simulink model "MASTER"  (R2019a)
settings: Solver=FixedStepAuto  StartTime=0.0  StopTime=10.0  FixedStep=0.001  RelTol=1e-3
PreLoadFcn:
  | waijung.modelPreload; % Required for working with Waijung Blockset. Do not remove.
undefined symbols (not defined in the file): HSEOSC, Link, LQFP100, ST, STM32F407VG
libraries: simulink x17, stm32f4_canbus_lib x7, stm32f4_tim_lib x1, stm32f4_io_lib x1, stm32f4_device_config_lib x1
(part 1 of 2)
CloseFcn:
  | waijung.modelClose; % Required for working with Waijung Blockset. Do not remove.
settings Model: Creator=Le Thanh Tu  LastModifiedBy=Le Thanh Tu
settings OptimizationCC: DefaultParameterBehavior=Inlined  PassReuseOutputArgsAs=Individual arguments
settings DebuggingCC: ParameterTunabilityLossMsg=error
settings HardwareCC: ProdBitPerPointer=32  ProdBitPerSizeT=32  ProdBitPerPtrDiffT=32  ProdLargestAtomicFloat=None  ProdIntDivRoundTo=Undefined  ProdWordSize=32  ProdHWDeviceType=ARM Compatible->Cortex - M4  TargetEndianess=LittleEndian  TargetHWDeviceType=ARM Compatible->Cortex - M4
settings SFSimCC: MATLABDynamicMemAlloc=off
settings RTWCC: SystemTargetFile=stm32f4.tlc  GenerateMakefile=off  TemplateMakefile=ert_default_tmf  Description=STM32F4 Target  GenerateReport=on  IncludeHyperlinkInReport=on  LaunchReport=on  GenerateTraceInfo=on  GenerateTraceReport=on  GenerateTraceReportSl=on  GenerateTraceReportSf=on  GenerateTraceReportEml=on
settings CodeAppCC: ForceParamTrailComments=on  IgnoreCustomStorageClasses=off  OperatorAnnotations=on  SimulinkDataObjDesc=on  SFDataObjDesc=on  InsertBlockDesc=on
settings STFCustomTargetCC: MultiwordLength=256  ModelReferenceCompliant=off  CombineOutputUpdateFcns=on  ERTCustomFileBanners=on  SupportNonInlinedSFcns=off  RemoveResetFunc=on  SupportVariableSizeSignals=on  MATLABClassNameForMDSCustomization=Simulink.SoftwareTarget.ERTCustomization  GRTInterface=off  SystemTargetFile=stm32f4.tlc
settings ERTTargetCC: ModelReferenceCompliant=off  ParMdlRefBuildCompliant=off  CompOptLevelCompliant=off  ConcurrentExecutionCompliant=off  SupportContinuousTime=on  SupportVariableSizeSignals=on  ModelStepFunctionPrototypeControlCompliant=off  CPPClassGenCompliant=off  UseToolchainInfoCompliant=off  InlinedParameterPlacement=NonHierarchical  ERTSrcFileBannerTemplate=stm32f4_code_template.cgt  ERTHdrFileBannerTemplate=stm32f4_code_template.cgt  ERTDataSrcFileTemplate=stm32f4_code_template.cgt  ERTDataHdrFileTemplate=stm32f4_code_template.cgt  ERTCustomFileTemplate=stm32f4_file_process.tlc

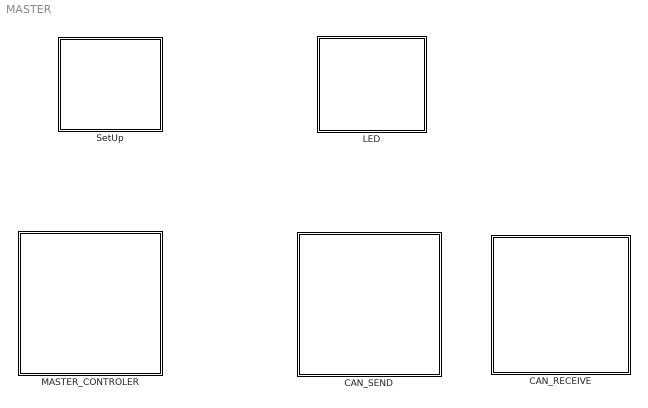
== system MASTER ==
  CAN_RECEIVE : Subsystem
  CAN_SEND : Subsystem
  LED : Subsystem
  MASTER_CONTROLER : Subsystem
  SetUp : Subsystem

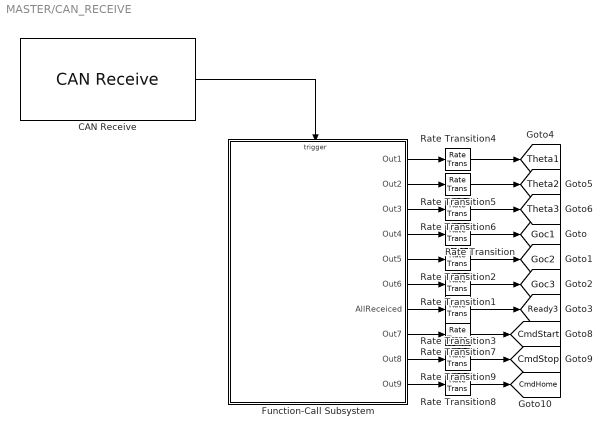
== system MASTER/CAN_RECEIVE ==
  CAN Receive : stm32f4_canbus_lib/CAN Receive  conf=Rx  canmodule=1  idtype=Standard  filtertype=Mask  id=0  idmask=0  enableisr=on  usedlc=off  datatype=single  data0type=uint32  data1type=uint32  data2type=Not used  data3type=Not used  data4type=Not used  data5type=Not used  data6type=Not used  data7type=Not used  buffersize=8  sampletime=-1  sampletimestr=-1  blockid=CAN_RECEIVECANReceive  inputarray=[]  inputlabelarray={}  outputarray=[7]  outputlabelarray={'Call ISR' }  compat=0  confstr="[\"Standard\",\"Mask\",\"0\",\"0\",\"off\",\"uint32\",\"uint32\",\"Not used\",\"Not used\",\"Not used\",\"Not used\",\"Not used\",\"Not used\",\"8\",\"0\",\"0\",\"0\",\"4\"]"
      settings: SourceProductName=Waijung Blockset
  Function-Call Subsystem : Subsystem  TreatAsAtomicUnit=on
  Rate Transition{,1..9} (10 alike) : RateTransition  Deterministic=off
  tag scope: CmdHome=global, CmdStart=global, CmdStop=global, Goc1=global, Goc2=global, Goc3=global, Ready3=global, Theta1=global, Theta2=global, Theta3=global
  wires:
  Function-Call Subsystem/7(AllReceiced) -> Rate Transition3/1
  Rate Transition2/1 -> [Goc2]
  Function-Call Subsystem/8(Out7) -> Rate Transition7/1
  Rate Transition1/1 -> [Goc3]
  CAN Receive/1 -> Function-Call Subsystem/Trigger
  Rate Transition/1 -> [Goc1]
  Rate Transition9/1 -> [CmdStop]
  Function-Call Subsystem/10(Out9) -> Rate Transition8/1
  Function-Call Subsystem/3(Out3) -> Rate Transition6/1
  Function-Call Subsystem/2(Out2) -> Rate Transition5/1
  Function-Call Subsystem/4(Out4) -> Rate Transition/1
  Rate Transition7/1 -> [CmdStart]
  Function-Call Subsystem/6(Out6) -> Rate Transition1/1
  Rate Transition6/1 -> [Theta3]
  Rate Transition3/1 -> [Ready3]
  Function-Call Subsystem/9(Out8) -> Rate Transition9/1
  Function-Call Subsystem/5(Out5) -> Rate Transition2/1
  Rate Transition8/1 -> [CmdHome]
  Rate Transition4/1 -> [Theta1]
  Rate Transition5/1 -> [Theta2]
  Function-Call Subsystem/1(Out1) -> Rate Transition4/1

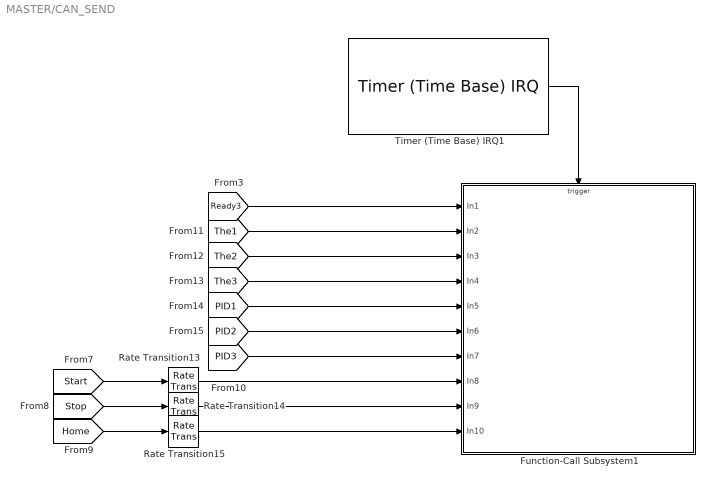
== system MASTER/CAN_SEND ==
  Function-Call Subsystem1 : Subsystem  TreatAsAtomicUnit=on
  Rate Transition13 : RateTransition  Deterministic=off
  Rate Transition14 : RateTransition  Deterministic=off
  Rate Transition15 : RateTransition  Deterministic=off
  Timer (Time Base) IRQ1 : stm32f4_tim_lib/Timer (Time Base) IRQ  configmode=Advance  timer=10  nvicprioritygroup=4  irqpreemptionpriority_g0=0  irqpreemptionpriority_g1=0  irqpreemptionpriority_g2=0  irqpreemptionpriority_g3=4  irqpreemptionpriority_g4=0  irqpreemptionpriority=0  irqsubpriority_g0=0  irqsubpriority_g1=0  irqsubpriority_g2=0  irqsubpriority_g3=0  irqsubpriority_g4=0  irqsubpriority=0  sampletime=0.01  autoreload=64614  prescaler=25  blockid=CAN_SENDTimerTimeBaseIRQ1
      settings: SourceProductName=Waijung Blockset
  wires:
  [The3] -> Function-Call Subsystem1/4(In4)
  [PID1] -> Function-Call Subsystem1/5(In5)
  Rate Transition14/1 -> Function-Call Subsystem1/9(In9)
  [Start] -> Rate Transition13/1
  [The1] -> Function-Call Subsystem1/2(In2)
  Rate Transition13/1 -> Function-Call Subsystem1/8(In8)
  [PID3] -> Function-Call Subsystem1/7(In7)
  [The2] -> Function-Call Subsystem1/3(In3)
  [Ready3] -> Function-Call Subsystem1/1(In1)
  [PID2] -> Function-Call Subsystem1/6(In6)
  Rate Transition15/1 -> Function-Call Subsystem1/10(In10)
  Timer (Time Base) IRQ1/1 -> Function-Call Subsystem1/Trigger
  [Home] -> Rate Transition15/1
  [Stop] -> Rate Transition14/1

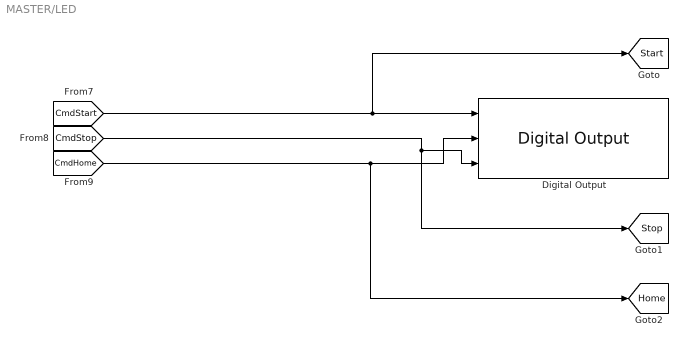
== system MASTER/LED ==
  Digital Output : stm32f4_io_lib/Digital Output  use_bitband=on  port=D  speed=100  porttype=Push Pull  porttypestr=PP  use_pin0=off  use_pin1=off  use_pin2=off  use_pin3=off  use_pin4=off  use_pin5=off  use_pin6=off  use_pin7=off  use_pin8=off  use_pin9=off  use_pin10=off  use_pin11=off  use_pin12=off  use_pin13=on  use_pin14=on  use_pin15=on  pinstr=GPIO_Pin_13 | GPIO_Pin_14 | GPIO_Pin_15  usedpinarray="[0  0  0  0  0  0  0  0  0  0  0  0  0  1  1  1]"  bitbandingstr=|  sampletime=-1  sampletimestr=-1  blockid=LEDDigitalOutput  enablecustomportlabel=off  globalinit=on  cinputportlabel=In1, In2  coutputportlabel=0
      | #define LEDDigitalOutput_D13 Peripheral_BB(GPIOD->ODR, 13)  /* Output pin */
      | #define LEDDigitalOutput_D14 Peripheral_BB(GPIOD->ODR, 14)  /* Output pin */
      | #define LEDDigitalOutput_D15 Peripheral_BB(GPIOD->ODR, 15)  /* Output pin */
      settings: SourceProductName=Waijung Blockset
  tag scope: Home=global, Start=global, Stop=global
  wires:
  [CmdStart] -> [Start], Digital Output/1
  [CmdStop] -> Digital Output/3, [Stop]
  [CmdHome] -> [Home], Digital Output/2

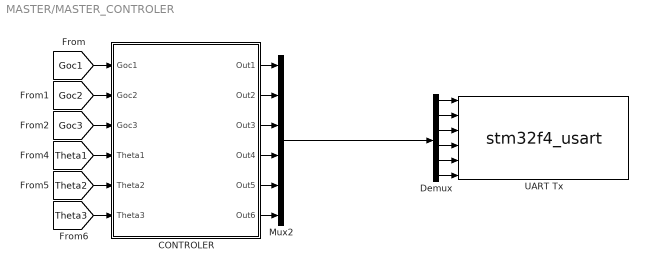
== system MASTER/MASTER_CONTROLER ==
  CONTROLER : Subsystem
  Demux : Demux  Outputs=6
  Mux2 : Mux  Inputs=6
  UART Tx : S-Function  Priority=1  FunctionName=stm32f4_usart  Parameters=configuration,uartmodule,transfer,baudrate,inputtype,outputtype,confstr,binheaderarray,binterminatorarray,asciiheader,asciiterminator,bindatalength,packetmode,varname,sampletime,sampletimestr,blockid  SFunctionDeploymentMode=off  EnableBusSupport=off  mask(stm32f4_usart){configuration=Tx, uartmodule=2, baudrate=115200, databits=8, parity=No, stopbit=1, remaptxpin=Not used, remaprxpin=Not used, flowcontrol=None, remapctspin=Not used, remaprtspin=Not used, advanceoptions=off, rxbuffersize=512, txbuffersize=512, transfer=Blocking, packetmode=Ascii, binheader='7E 7E', binterminator='03 03', porttype_double=1, porttype_single=0, porttype_int8=1, porttype_uint8=0, porttype_int16=0, porttype_uint16=0, porttype_int32=0, porttype_uint32=0, asciiformat='%f, %f, %f, %f, %f, %f', rx_asciiterminator=CRLF (0x0D 0x0A - "\r\n"), tx_asciiterminator=CRLF (0x0D 0x0A - "\r\n"), storagename=<empty>, varname=, inputtype=[6  1 1 1 1 1 1], outputtype=[0], binheaderarray=[0], binterminatorarray=[0], bindatalength=0, asciiheader='%f, %f, %f, %f, %f, %f\r\n', asciiterminator=[2 13 10], sampletime=0.01, sampletimestr=-1, blockid=MASTER_CONTROLERUARTTx, confstr=[ "dummy", "0", "*", "*", "0", "*", "*", "0", "*", "*", "0", "*", "*", "1", "4", "6", "1", "4", "5", "512", "512", "1", "2", "115200", "8", "No", "1", "None", "USART2"], lastmodule=1}
      mask prompts: uartmodule "UART Module"; baudrate "Baud rate (bps)"; databits "Data bits"; stopbit "Stop bit"; remaptxpin "Tx Pin"; remaprxpin "Rx Pin"; flowcontrol "Hardware flow control"; remapctspin "HW Flow control, CTS Pin"; remaprtspin "HW Flow control, RTS Pin"; advanceoptions "Advance options"; rxbuffersize "Rx buffer size (bytes)"; txbuffersize "Tx buffer size (bytes)"; packetmode "Packet mode"; binheader "Binary header (example: '7E 7E')"; binterminator "Binary terminator (example: '03 03')"; porttype_double "Number of data port, type DOUBLE"; porttype_single "Number of data port, type SINGLE"; porttype_int8 "Number of data port, type INT8"; porttype_uint8 "Number of data port, type UINT8"; porttype_int16 "Number of data port, type INT16"; porttype_uint16 "Number of data port, type UINT16"; porttype_int32 "Number of data port, type INT32"; porttype_uint32 "Number of data port, type UINT32"; asciiformat "Ascii format"; rx_asciiterminator "End of packet"; tx_asciiterminator "End of packet"; storagename "Buffer"; varname "Var name"; inputtype "Input data type"; outputtype "Output data type"; binheaderarray "Binary header"; binterminatorarray "Binary terminator"; bindatalength "Binary data length"; asciiheader "Ascii header (printf format)"; asciiterminator "Ascii terminator"; sampletime "Sample time (sec)"; sampletimestr "Compiled sample time (sec) in string"; confstr "Configuration string"; lastmodule "Last module selected"
      mask help:
      | Data type for Ascii format
      | %u, %i, %d, %o, %x: uint32
      | %e, %g, %f: single
      | %c: int8
      mask init:
      | stm32f4_usart_callback('init');
      mask Help: web(fullfile(waijungdocroot,'stm32f4_usart_tx.htm'), '-browser')
      mask TypeOptions configuration: Setup | Tx | Rx
      mask Callback configuration: stm32f4_usart_callback('configuration');
      mask TypeOptions uartmodule: 1 | 2 | 3 | 4 | 5 | 6
      mask Callback uartmodule: stm32f4_usart_callback('uartmodule');
      mask Callback baudrate: stm32f4_usart_callback('baudrate');
      mask TypeOptions databits: 8
      mask TypeOptions parity: No | Odd | Even
      mask TypeOptions stopbit: 0.5 | 1 | 1.5 | 2
      mask TypeOptions remaptxpin: Not used | A9 | B6
      mask TypeOptions remaprxpin: Not used | A10 | B7
      mask TypeOptions flowcontrol: None | RTS | CTS | RTS/CTS
      mask Callback flowcontrol: stm32f4_usart_callback('flowcontrol');
      mask TypeOptions remapctspin: Not used | A11
      mask TypeOptions remaprtspin: Not used | A12
      mask Callback advanceoptions: stm32f4_usart_callback('advanceoptions');
      mask TypeOptions rxbuffersize: 16 | 32 | 64 | 128 | 256 | 512 | 1024 | 2048
      mask TypeOptions txbuffersize: 16 | 32 | 64 | 128 | 256 | 512 | 1024 | 2048
      mask TypeOptions transfer: Blocking | Non-Blocking
      mask Callback transfer: stm32f4_usart_callback('transfer');
      mask TypeOptions packetmode: Ascii | Binary | Binary Vector | String Buffer | Raw Buffer
      mask Callback packetmode: stm32f4_usart_callback('packetmode');
      mask Callback binheader: stm32f4_usart_callback('binheader');
      mask Callback binterminator: stm32f4_usart_callback('binterminator');
      mask Callback porttype_double: stm32f4_usart_callback('porttype');
      mask Callback porttype_single: stm32f4_usart_callback('porttype');
      mask Callback porttype_int8: stm32f4_usart_callback('porttype');
      mask Callback porttype_uint8: stm32f4_usart_callback('porttype');
      mask Callback porttype_int16: stm32f4_usart_callback('porttype');
      mask Callback porttype_uint16: stm32f4_usart_callback('porttype');
      mask Callback porttype_int32: stm32f4_usart_callback('porttype');
      mask Callback porttype_uint32: stm32f4_usart_callback('porttype');
      mask Callback asciiformat: stm32f4_usart_callback('asciiformat');
      mask TypeOptions rx_asciiterminator: CR (0x0D - "\r") | LF (0x0A - "\n") | CRLF (0x0D 0x0A - "\r\n")
      mask Callback rx_asciiterminator: stm32f4_usart_callback('rx_asciiterminator');
      mask TypeOptions tx_asciiterminator: CR (0x0D - "\r") | LF (0x0A - "\n") | CRLF (0x0D 0x0A - "\r\n") | None
      mask Callback tx_asciiterminator: stm32f4_usart_callback('tx_asciiterminator');
      mask TypeOptions storagename: <empty>
      mask Callback storagename: stm32f4_usart_callback('storagename');
      mask Callback varname: stm32f4_usart_callback('varname');
      mask Callback sampletime: stm32f4_usart_callback('sampletime');
      mask Callback sampletimestr: stm32f4_usart_callback('sampletimestr');
      mask Callback blockid: stm32f4_usart_callback('blockid');
      mask Display: text(0.95, 0.5, 'Module: USART2_Tx\nPacket: Ascii\nTransfer: Blocking\nTs (sec): -1','ver','middle','hor','right'); port_label('input', 1,'single'); port_label('input', 2,'single'); port_label('input', 3,'single'); port_label('input', 4,'single'); port_label('input', 5,'single'); port_label('input', 6,'single');
  wires:
  CONTROLER/4(Out4) -> Mux2/4
  CONTROLER/6(Out6) -> Mux2/6
  Demux/1 -> UART Tx/1
  Demux/4 -> UART Tx/4
  Demux/3 -> UART Tx/3
  Demux/5 -> UART Tx/5
  CONTROLER/5(Out5) -> Mux2/5
  Mux2/1 -> Demux/1
  Demux/2 -> UART Tx/2
  Demux/6 -> UART Tx/6
  CONTROLER/1(Out1) -> Mux2/1
  [Goc3] -> CONTROLER/3(Goc3)
  [Theta1] -> CONTROLER/4(Theta1)
  [Theta2] -> CONTROLER/5(Theta2)
  [Goc1] -> CONTROLER/1(Goc1)
  [Goc2] -> CONTROLER/2(Goc2)
  CONTROLER/2(Out2) -> Mux2/2
  [Theta3] -> CONTROLER/6(Theta3)
  CONTROLER/3(Out3) -> Mux2/3

== system MASTER/SetUp ==
  CAN Setup1 : S-Function  FunctionName=stm32f4_can  Parameters=conf,canmodule,0,inputarray,outputarray,'','',confstr,sampletime,sampletimestr,blockid  SFunctionDeploymentMode=off  EnableBusSupport=off  mask(stm32f4_can){conf=Setup, canmodule=1, advance=on, bitrate_select=125000, sjw=1tq, bs1=3tq, bs2=2tq, timingconf=Prescaler, brp=7, bitrate=1000000, tq=1.6667e-07, autoretransmission=Enable, remaptxpin=B9, remaprxpin=B8, sampletime=-1, sampletimestr=-1, blockid=SetUpCANSetup1, inputarray=[], inputlabelarray={}, outputarray=[], outputlabelarray={}, compat=0, confstr=["1000000","7","B","9","B","8","1tq","3tq","2tq","DISABLE"], presc=7, txportstr=B, txpinstr=9, rxportstr=B, rxpinstr=8, lastmodule=1}
      mask prompts: conf "Configuration"; canmodule "CAN Module"; advance "Advance configuration"; bitrate_select "Baud rate (bps)"; sjw "Resync Jump Width (SJW)"; bs1 "Bit segment 1 (BS1) + PROP_SEG"; bs2 "Bit segment 2 (BS2)"; timingconf "Adjust"; brp "Baud rate prescaler (BRP)"; bitrate "Baud rate (bps)"; tq "Time Quantum (Second), tq"; autoretransmission "Auto Re-transmission"; remaptxpin "CAN Tx pin"; remaprxpin "CAN Rx pin"; sampletime "Sample time (sec)"; sampletimestr "Compiled sample time (sec) in string"; inputarray "Input port"; inputlabelarray "Input port label"; outputarray "Output port"; outputlabelarray "Output port label"; compat "Compatibility (Reserved for future use)"; confstr "Configuration String"; presc "Prescale"; txportstr "Tx port string"; txpinstr "Tx pin string"; rxportstr "Rx port string"; rxpinstr "Rx pin string"; lastmodule "Last module selected"
      mask help:
      | This block setups CAN Module.
      |
      | Auto Re-transmission,
      |  - Enable: The CAN hardware will automatically retransmit the message until it has been
      | successfully transmitted according to the CAN standard.
      |  - Disable: A message will be transmitted only once, independently of the transmission result
      | (successful, error or arbitration lost).
      mask init:
      | stm32f4_can_callback('init');
      mask Help: web(fullfile(waijungdocroot,'stm32f4_can_setup.htm'), '-browser')
      mask TypeOptions conf: Setup
      mask TypeOptions canmodule: 1 | 2
      mask Callback canmodule: stm32f4_can_callback('canmodule');
      mask Callback advance: stm32f4_can_callback('advance');
      mask TypeOptions bitrate_select: 125000 | 250000 | 500000 | 1000000
      mask Callback bitrate_select: stm32f4_can_callback('bitrate_select');
      mask TypeOptions sjw: 1tq | 2tq | 3tq | 4tq
      mask TypeOptions bs1: 1tq | 2tq | 3tq | 4tq | 5tq | 6tq | 7tq | 8tq | 9tq | 10tq | 11tq | 12tq | 13tq | 14tq | 15tq | 16tq
      mask Callback bs1: stm32f4_can_callback('timingconf');
      mask TypeOptions bs2: 1tq | 2tq | 3tq | 4tq | 5tq | 6tq | 7tq | 8tq
      mask Callback bs2: stm32f4_can_callback('timingconf');
      mask TypeOptions timingconf: Prescaler | Baudrate
      mask Callback timingconf: stm32f4_can_callback('timingconf');
      mask Callback brp: stm32f4_can_callback('timingconf');
      mask Callback bitrate: stm32f4_can_callback('timingconf');
      mask TypeOptions autoretransmission: Enable | Disable
      mask TypeOptions remaptxpin: Not used | A12 | B9 | D1
      mask Callback remaptxpin: stm32f4_can_callback('remaptxpin');
      mask TypeOptions remaprxpin: Not used | A11 | B8 | D0
      mask Callback remaprxpin: stm32f4_can_callback('remaprxpin');
      mask Callback sampletime: stm32f4_can_callback('sampletime');
      mask Callback sampletimestr: stm32f4_can_callback('sampletimestr');
      mask Callback blockid: stm32f4_can_callback('blockid');
      mask Display: text(0.5, 0.5, 'CAN1_Setup\nSpeed (bps): 1000000\nTx/Rx pin: B9/B8','ver','middle','hor','center');
  Target Setup : stm32f4_device_config_lib/Target Setup  Priority=100  compiler=GNU ARM  previous_compiler=GNU ARM  mcu=STM32F407VG (LQFP100)  mcustr=STM32F407VG  clockconfig=HSEOSC-8MHz  system_stm32f4xx_c_path=D:\fix_waijung\waijung17_03a\waijung17_03a\targets\stm32f4_target\stm32f4\utils\system_stm32f4xx_default\STM32F40_41xxx\hseosc8mhz  showmemoryconfiguration=off  stacksize=0x2000  heapsize=0x2000  enableautocompiledownload=on  fullchiperase=off  programmerinterface=ST-Link  editctrlstr=on  compilercontrolstr=$(patsubst %, -I%, .) -mcpu=cortex-m4 -mthumb -mthumb-interwork -mfloat-abi=hard -mfpu=fpv4-sp-d16 -ffast-math -Wall -Wextra -Ofast  assemblercontrolstr=$(patsubst %, -I%, .) -mcpu=cortex-m4 -mthumb -mthumb-interwork -mfloat-abi=hard -mfpu=fpv4-sp-d16 -ffast-math -Wall -Wextra -Ofast -Wa,-amhls=$(<:.s=.lst) -D__STACK_SIZE=$(STACK_SIZE) -D__HEAP_SIZE=$(HEAP_SIZE)  linkercontrolstr=-T$(LD_SCRIPT) -g -Wl,-Map=$(MAP),--cref,--no-warn-mismatch -mcpu=cortex-m4 -mthumb -mthumb-interwork -mfloat-abi=hard -mfpu=fpv4-sp-d16 -specs=nosys.specs  runafterdownload=on  execprofile=Real-time output  profileruart=3  profilerbaud=500000  profilertxpin=D8  profilerinitstr=0.001,168000000,168000,500000,0  manualsetsampletime=on  sampletime=0.001  blockid=SetUpTargetSetup  systickreloadvalue=168000  hseval=8000000  lastprofileruart=3  hclk=168000000  flashorigin=0x8000000  flashlength=1024k  ramorigin=0x20000000  ramlength=128k  useextram=off
      settings: SourceProductName=Waijung Blockset
  UART Setup : S-Function  Priority=1  FunctionName=stm32f4_usart  Parameters=configuration,uartmodule,transfer,baudrate,inputtype,outputtype,confstr,binheaderarray,binterminatorarray,asciiheader,asciiterminator,bindatalength,packetmode,varname,sampletime,sampletimestr,blockid  SFunctionDeploymentMode=off  EnableBusSupport=off  mask(stm32f4_usart){configuration=Setup, uartmodule=2, baudrate=115200, databits=8, parity=No, stopbit=1, remaptxpin=A2, remaprxpin=A3, flowcontrol=None, remapctspin=Not used, remaprtspin=Not used, advanceoptions=on, rxbuffersize=512, txbuffersize=512, transfer=Blocking, packetmode=Ascii, binheader='7E 7E', binterminator='03 03', porttype_double=1, porttype_single=0, porttype_int8=1, porttype_uint8=0, porttype_int16=0, porttype_uint16=0, porttype_int32=0, porttype_uint32=0, asciiformat='%d,%f', rx_asciiterminator=CRLF (0x0D 0x0A - "\r\n"), tx_asciiterminator=CR (0x0D - "\r"), storagename=<empty>, varname=, inputtype=[0], outputtype=[0], binheaderarray=[0], binterminatorarray=[0], bindatalength=0, asciiheader='', asciiterminator=[0], sampletime=-1, sampletimestr=-1, blockid=SetUpUARTSetup, confstr=[ "dummy", "1", "A", "2", "1", "A", "3", "0", "*", "*", "0", "*", "*", "1", "4", "6", "1", "4", "5", "512", "512", "1", "2", "115200", "8", "No", "1", "None", "USART2"], lastmodule=2}
      mask prompts: uartmodule "UART Module"; baudrate "Baud rate (bps)"; databits "Data bits"; stopbit "Stop bit"; remaptxpin "Tx Pin"; remaprxpin "Rx Pin"; flowcontrol "Hardware flow control"; remapctspin "HW Flow control, CTS Pin"; remaprtspin "HW Flow control, RTS Pin"; advanceoptions "Advance options"; rxbuffersize "Rx buffer size (bytes)"; txbuffersize "Tx buffer size (bytes)"; packetmode "Packet mode"; binheader "Binary header (example: '7E 7E')"; binterminator "Binary terminator (example: '03 03')"; porttype_double "Number of data port, type DOUBLE"; porttype_single "Number of data port, type SINGLE"; porttype_int8 "Number of data port, type INT8"; porttype_uint8 "Number of data port, type UINT8"; porttype_int16 "Number of data port, type INT16"; porttype_uint16 "Number of data port, type UINT16"; porttype_int32 "Number of data port, type INT32"; porttype_uint32 "Number of data port, type UINT32"; asciiformat "Ascii format"; rx_asciiterminator "End of packet"; tx_asciiterminator "End of packet"; storagename "Buffer"; varname "Var name"; inputtype "Input data type"; outputtype "Output data type"; binheaderarray "Binary header"; binterminatorarray "Binary terminator"; bindatalength "Binary data length"; asciiheader "Ascii header (printf format)"; asciiterminator "Ascii terminator"; sampletime "Sample time (sec)"; sampletimestr "Compiled sample time (sec) in string"; confstr "Configuration string"; lastmodule "Last module selected"
      mask help:
      | Default STM32F4DISCOVERY + aMG F4 Connect 2 + aMG USB Converter N2 settings use
      |
      | USART3, Tx D8, Rx D9 and USB Serial Converter A.
      mask init:
      | stm32f4_usart_callback('init');
      mask Help: web(fullfile(waijungdocroot,'stm32f4_usart_setup.htm'), '-browser')
      mask TypeOptions configuration: Setup | Tx | Rx
      mask Callback configuration: stm32f4_usart_callback('configuration');
      mask TypeOptions uartmodule: 1 | 2 | 3 | 4 | 5 | 6
      mask Callback uartmodule: stm32f4_usart_callback('uartmodule');
      mask Callback baudrate: stm32f4_usart_callback('baudrate');
      mask TypeOptions databits: 8
      mask TypeOptions parity: No | Odd | Even
      mask TypeOptions stopbit: 0.5 | 1 | 1.5 | 2
      mask TypeOptions remaptxpin: Not used | A2 | D5
      mask TypeOptions remaprxpin: Not used | A3 | D6
      mask TypeOptions flowcontrol: None | RTS | CTS | RTS/CTS
      mask Callback flowcontrol: stm32f4_usart_callback('flowcontrol');
      mask TypeOptions remapctspin: Not used | A0 | D3
      mask TypeOptions remaprtspin: Not used | A1 | D4
      mask Callback advanceoptions: stm32f4_usart_callback('advanceoptions');
      mask TypeOptions rxbuffersize: 16 | 32 | 64 | 128 | 256 | 512 | 1024 | 2048
      mask TypeOptions txbuffersize: 16 | 32 | 64 | 128 | 256 | 512 | 1024 | 2048
      mask TypeOptions transfer: Blocking | Non-Blocking
      mask Callback transfer: stm32f4_usart_callback('transfer');
      mask TypeOptions packetmode: Ascii | Binary | String Buffer
      mask Callback packetmode: stm32f4_usart_callback('packetmode');
      mask Callback binheader: stm32f4_usart_callback('binheader');
      mask Callback binterminator: stm32f4_usart_callback('binterminator');
      mask Callback porttype_double: stm32f4_usart_callback('porttype');
      mask Callback porttype_single: stm32f4_usart_callback('porttype');
      mask Callback porttype_int8: stm32f4_usart_callback('porttype');
      mask Callback porttype_uint8: stm32f4_usart_callback('porttype');
      mask Callback porttype_int16: stm32f4_usart_callback('porttype');
      mask Callback porttype_uint16: stm32f4_usart_callback('porttype');
      mask Callback porttype_int32: stm32f4_usart_callback('porttype');
      mask Callback porttype_uint32: stm32f4_usart_callback('porttype');
      mask Callback asciiformat: stm32f4_usart_callback('asciiformat');
      mask TypeOptions rx_asciiterminator: CR (0x0D - "\r") | LF (0x0A - "\n") | CRLF (0x0D 0x0A - "\r\n")
      mask Callback rx_asciiterminator: stm32f4_usart_callback('rx_asciiterminator');
      mask TypeOptions tx_asciiterminator: CR (0x0D - "\r") | LF (0x0A - "\n") | CRLF (0x0D 0x0A - "\r\n") | None
      mask Callback tx_asciiterminator: stm32f4_usart_callback('tx_asciiterminator');
      mask TypeOptions storagename: <empty>
      mask Callback storagename: stm32f4_usart_callback('storagename');
      mask Callback varname: stm32f4_usart_callback('varname');
      mask Callback sampletime: stm32f4_usart_callback('sampletime');
      mask Callback sampletimestr: stm32f4_usart_callback('sampletimestr');
      mask Callback blockid: stm32f4_usart_callback('blockid');
      mask Display: text(0.5, 0.5, 'Module: USART2_Setup\nBaud (Bps): 115200\nDMA Buffer: 512/512\nTx/Rx Pin: A2/A3','ver','middle','hor','center');

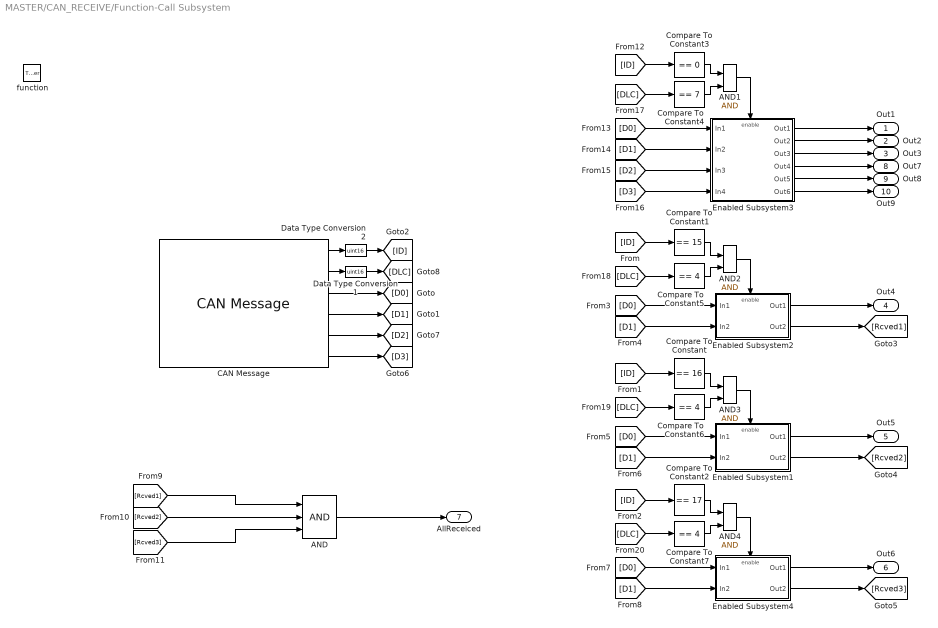
== system MASTER/CAN_RECEIVE/Function-Call Subsystem ==
  function : TriggerPort  TriggerType=function-call  VariantControl=Variant
  AND : Logic  Inputs=3  IconShape=distinctive  AllPortsSameDT=off  OutDataTypeStr=boolean
  AND{1..4} (4 alike) : Logic  IconShape=distinctive  AllPortsSameDT=off  OutDataTypeStr=boolean
  CAN Message : stm32f4_canbus_lib/CAN Message  conf=Msg  canmodule=1  usedlc=on  datatype=double  data0type=int16  data1type=int16  data2type=int16  data3type=uint8  data4type=Not used  data5type=Not used  data6type=Not used  data7type=Not used  sampletime=-1  sampletimestr=-1  blockid=CAN_RECEIVEFunctionCallSubsystemCANMessage  inputarray=[]  inputlabelarray={}  outputarray=[ 7, 3, 4, 4, 4, 3]  outputlabelarray={'ID','DLC', 'D0 (int16)', 'D1 (int16)', 'D2 (int16)', 'D3 (uint8)' }  compat=0  confstr="[\"on\",\"int16\",\"int16\",\"int16\",\"uint8\",\"Not used\",\"Not used\",\"Not used\",\"Not used\"]"
      settings: SourceProductName=Waijung Blockset
  Compare To Constant : simulink/Logic and Bit Operations/Compare To Constant  relop===  const=16  OutDataTypeStr=boolean
  Compare To Constant1 : simulink/Logic and Bit Operations/Compare To Constant  relop===  const=15  OutDataTypeStr=boolean
  Compare To Constant2 : simulink/Logic and Bit Operations/Compare To Constant  relop===  const=17  OutDataTypeStr=boolean
  Compare To Constant3 : simulink/Logic and Bit Operations/Compare To Constant  relop===  const=0  OutDataTypeStr=boolean
  Compare To Constant4 : simulink/Logic and Bit Operations/Compare To Constant  relop===  const=7  OutDataTypeStr=boolean
  Compare To Constant5 : simulink/Logic and Bit Operations/Compare To Constant  relop===  const=4  OutDataTypeStr=boolean
  Compare To Constant6 : simulink/Logic and Bit Operations/Compare To Constant  relop===  const=4  OutDataTypeStr=boolean
  Compare To Constant7 : simulink/Logic and Bit Operations/Compare To Constant  relop===  const=4  OutDataTypeStr=boolean
  Data Type Conversion1 : DataTypeConversion  OutDataTypeStr=uint16
  Data Type Conversion2 : DataTypeConversion  OutDataTypeStr=uint16
  Enabled Subsystem1 : Subsystem  TreatAsAtomicUnit=on
  Enabled Subsystem2 : Subsystem  TreatAsAtomicUnit=on
  Enabled Subsystem3 : Subsystem  TreatAsAtomicUnit=on
  Enabled Subsystem4 : Subsystem  TreatAsAtomicUnit=on
  Out1 : Outport
  Out2 : Outport  Port=2
  Out3 : Outport  Port=3
  Out4 : Outport  Port=4
  Out5 : Outport  Port=5
  Out6 : Outport  Port=6
  AllReceiced : Outport  Port=7
  Out7 : Outport  Port=8
  Out8 : Outport  Port=9
  Out9 : Outport  Port=10
  wires:
  [D0] -> Enabled Subsystem4/1(In1)
  CAN Message/1 -> Data Type Conversion2/1
  Data Type Conversion2/1 -> [ID]
  [ID] -> Compare To Constant1/1
  [ID] -> Compare To Constant/1
  [ID] -> Compare To Constant2/1
  Enabled Subsystem2/2(Out2) -> [Rcved1]
  Enabled Subsystem1/2(Out2) -> [Rcved2]
  [D1] -> Enabled Subsystem4/2(In2)
  Enabled Subsystem4/2(Out2) -> [Rcved3]
  [D0] -> Enabled Subsystem2/1(In1)
  [D1] -> Enabled Subsystem2/2(In2)
  [D0] -> Enabled Subsystem1/1(In1)
  [D1] -> Enabled Subsystem1/2(In2)
  [D1] -> Enabled Subsystem3/2(In2)
  [D0] -> Enabled Subsystem3/1(In1)
  Enabled Subsystem3/2(Out2) -> Out2/1
  [ID] -> Compare To Constant3/1
  Enabled Subsystem3/1(Out1) -> Out1/1
  [D2] -> Enabled Subsystem3/3(In3)
  Enabled Subsystem3/3(Out3) -> Out3/1
  Enabled Subsystem2/1(Out1) -> Out4/1
  Enabled Subsystem1/1(Out1) -> Out5/1
  Enabled Subsystem4/1(Out1) -> Out6/1
  [D3] -> Enabled Subsystem3/4(In4)
  Enabled Subsystem3/4(Out4) -> Out7/1
  Enabled Subsystem3/5(Out5) -> Out8/1
  Enabled Subsystem3/6(Out6) -> Out9/1
  CAN Message/3 -> [D0]
  CAN Message/4 -> [D1]
  CAN Message/5 -> [D2]
  CAN Message/6 -> [D3]
  CAN Message/2 -> Data Type Conversion1/1
  Compare To Constant3/1 -> AND1/1
  [DLC] -> Compare To Constant4/1
  Compare To Constant4/1 -> AND1/2
  AND1/1 -> Enabled Subsystem3/Enable
  AND2/1 -> Enabled Subsystem2/Enable
  Compare To Constant5/1 -> AND2/2
  [DLC] -> Compare To Constant5/1
  Compare To Constant1/1 -> AND2/1
  AND3/1 -> Enabled Subsystem1/Enable
  Compare To Constant6/1 -> AND3/2
  [DLC] -> Compare To Constant6/1
  Compare To Constant/1 -> AND3/1
  AND4/1 -> Enabled Subsystem4/Enable
  Compare To Constant7/1 -> AND4/2
  [DLC] -> Compare To Constant7/1
  Compare To Constant2/1 -> AND4/1
  Data Type Conversion1/1 -> [DLC]
  AND/1 -> AllReceiced/1
  [Rcved1] -> AND/1
  [Rcved2] -> AND/2
  [Rcved3] -> AND/3

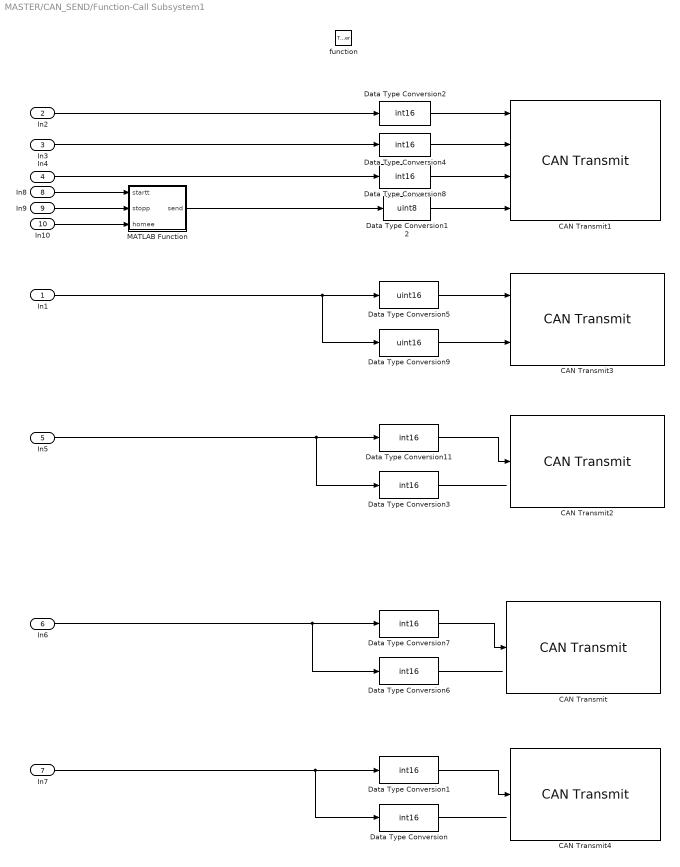
== system MASTER/CAN_SEND/Function-Call Subsystem1 ==
  In1 : Inport
  In2 : Inport  Port=2
  In3 : Inport  Port=3
  In4 : Inport  Port=4
  In5 : Inport  Port=5
  In6 : Inport  Port=6
  In7 : Inport  Port=7
  In8 : Inport  Port=8
  In9 : Inport  Port=9
  In10 : Inport  Port=10
  function : TriggerPort  TriggerType=function-call  VariantControl=Variant
  CAN Transmit : stm32f4_canbus_lib/CAN Transmit  conf=Tx  canmodule=1  transfer=Blocking  timeout=0.002  idtype=Standard  specificid=on  id=2043  specificdlc=on  dlc=2  enablestatus=off  datatype=single  data0type=int16  data1type=Not used  data2type=Not used  data3type=Not used  data4type=Not used  data5type=Not used  data6type=Not used  data7type=Not used  inputarray=[ 4]  inputlabelarray={ 'D0 (int16)' }  outputarray=[]  outputlabelarray={}  sampletime=-1  sampletimestr=-1  blockid=CAN_SENDFunctionCallSubsystem1CANTransmit  compat=0  confstr="[\"Blocking\",\"0.002\",\"Standard\",\"on\",\"2043\",\"on\",\"2\",\"off\",\"int16\",\"Not used\",\"Not used\",\"Not used\",\"Not used\",\"Not used\",\"Not used\",\"Not used\"]"
      settings: SourceProductName=Waijung Blockset
  CAN Transmit1 : stm32f4_canbus_lib/CAN Transmit  conf=Tx  canmodule=1  transfer=Blocking  timeout=0.004  idtype=Standard  specificid=on  id=1  specificdlc=on  dlc=7  enablestatus=off  datatype=single  data0type=int16  data1type=int16  data2type=int16  data3type=uint8  data4type=Not used  data5type=Not used  data6type=Not used  data7type=Not used  inputarray=[ 4, 4, 4, 3]  inputlabelarray={ 'D0 (int16)', 'D1 (int16)', 'D2 (int16)', 'D3 (uint8)' }  outputarray=[]  outputlabelarray={}  sampletime=-1  sampletimestr=-1  blockid=CAN_SENDFunctionCallSubsystem1CANTransmit1  compat=0  confstr="[\"Blocking\",\"0.004\",\"Standard\",\"on\",\"1\",\"on\",\"7\",\"off\",\"int16\",\"int16\",\"int16\",\"uint8\",\"Not used\",\"Not used\",\"Not used\",\"Not used\"]"
      settings: SourceProductName=Waijung Blockset
  CAN Transmit2 : stm32f4_canbus_lib/CAN Transmit  conf=Tx  canmodule=1  transfer=Blocking  timeout=0.0015  idtype=Standard  specificid=on  id=2039  specificdlc=on  dlc=2  enablestatus=off  datatype=single  data0type=int16  data1type=Not used  data2type=Not used  data3type=Not used  data4type=Not used  data5type=Not used  data6type=Not used  data7type=Not used  inputarray=[ 4]  inputlabelarray={ 'D0 (int16)' }  outputarray=[]  outputlabelarray={}  sampletime=-1  sampletimestr=-1  blockid=CAN_SENDFunctionCallSubsystem1CANTransmit2  compat=0  confstr="[\"Blocking\",\"0.0015\",\"Standard\",\"on\",\"2039\",\"on\",\"2\",\"off\",\"int16\",\"Not used\",\"Not used\",\"Not used\",\"Not used\",\"Not used\",\"Not used\",\"Not used\"]"
      settings: SourceProductName=Waijung Blockset
  CAN Transmit3 : stm32f4_canbus_lib/CAN Transmit  conf=Tx  canmodule=1  transfer=Blocking  timeout=0.001  idtype=Standard  specificid=on  id=2047  specificdlc=on  dlc=4  enablestatus=off  datatype=single  data0type=uint16  data1type=uint16  data2type=Not used  data3type=Not used  data4type=Not used  data5type=Not used  data6type=Not used  data7type=Not used  inputarray=[ 5, 5]  inputlabelarray={ 'D0 (uint16)', 'D1 (uint16)' }  outputarray=[]  outputlabelarray={}  sampletime=-1  sampletimestr=-1  blockid=CAN_SENDFunctionCallSubsystem1CANTransmit3  compat=0  confstr="[\"Blocking\",\"0.001\",\"Standard\",\"on\",\"2047\",\"on\",\"4\",\"off\",\"uint16\",\"uint16\",\"Not used\",\"Not used\",\"Not used\",\"Not used\",\"Not used\",\"Not used\"]"
      settings: SourceProductName=Waijung Blockset
  CAN Transmit4 : stm32f4_canbus_lib/CAN Transmit  conf=Tx  canmodule=1  transfer=Blocking  timeout=0.002  idtype=Standard  specificid=on  id=2045  specificdlc=on  dlc=2  enablestatus=off  datatype=single  data0type=int16  data1type=Not used  data2type=Not used  data3type=Not used  data4type=Not used  data5type=Not used  data6type=Not used  data7type=Not used  inputarray=[ 4]  inputlabelarray={ 'D0 (int16)' }  outputarray=[]  outputlabelarray={}  sampletime=-1  sampletimestr=-1  blockid=CAN_SENDFunctionCallSubsystem1CANTransmit4  compat=0  confstr="[\"Blocking\",\"0.002\",\"Standard\",\"on\",\"2045\",\"on\",\"2\",\"off\",\"int16\",\"Not used\",\"Not used\",\"Not used\",\"Not used\",\"Not used\",\"Not used\",\"Not used\"]"
      settings: SourceProductName=Waijung Blockset
  Data Type Conversion{,1..4,6..8,11} (9 alike) : DataTypeConversion  OutDataTypeStr=int16
  Data Type Conversion12 : DataTypeConversion  OutDataTypeStr=uint8
  Data Type Conversion5 : DataTypeConversion  OutDataTypeStr=uint16
  Data Type Conversion9 : DataTypeConversion  OutDataTypeStr=uint16
  MATLAB Function : MATLAB Function  TreatAsAtomicUnit=on
  wires:
  In1/1 -> Data Type Conversion9/1, Data Type Conversion5/1
  Data Type Conversion9/1 -> CAN Transmit3/2
  Data Type Conversion5/1 -> CAN Transmit3/1
  In2/1 -> Data Type Conversion2/1
  In3/1 -> Data Type Conversion4/1
  In4/1 -> Data Type Conversion8/1
  In6/1 -> Data Type Conversion6/1, Data Type Conversion7/1
  Data Type Conversion/1 -> ?
  In5/1 -> Data Type Conversion3/1, Data Type Conversion11/1
  Data Type Conversion11/1 -> CAN Transmit2/1
  Data Type Conversion7/1 -> CAN Transmit/1
  Data Type Conversion6/1 -> ?
  Data Type Conversion3/1 -> ?
  In7/1 -> Data Type Conversion1/1, Data Type Conversion/1
  MATLAB Function/1(send) -> Data Type Conversion12/1
  Data Type Conversion12/1 -> CAN Transmit1/4
  In8/1 -> MATLAB Function/1(startt)
  In9/1 -> MATLAB Function/2(stopp)
  In10/1 -> MATLAB Function/3(homee)
  Data Type Conversion2/1 -> CAN Transmit1/1
  Data Type Conversion4/1 -> CAN Transmit1/2
  Data Type Conversion8/1 -> CAN Transmit1/3
  Data Type Conversion1/1 -> CAN Transmit4/1
